simulink model "visualize_imu"  (Simulink 8.8)
settings: Solver=FixedStepDiscrete  StartTime=0.0  StopTime=inf  FixedStep=0.01  RelTol=1e-3  EnableMultiTasking=on
libraries: WBToolboxLibrary x2
settings Model: SuppressorTable=22 serialization::archive 11 0 3 0 0 0 11 0  Creator=The MathWorks, Inc.  LastModifiedBy=gnava
settings DataIOCC: SaveFormat=Dataset  SignalLoggingSaveFormat=Dataset
settings DebuggingCC: UnderspecifiedInitializationDetection=Simplified  MergeDetectMultiDrivingBlocksExec=error  FcnCallInpInsideContextMsg=error  AllowSymbolicDim=off  StateNameClashWarn=none
settings HardwareCC: ProdBitPerPointer=64  ProdBitPerSizeT=64  ProdBitPerPtrDiffT=64  ProdLargestAtomicFloat=Float  ProdIntDivRoundTo=Zero  ProdEndianess=LittleEndian  ProdWordSize=64  ProdHWDeviceType=Intel->x86-64 (Windows64)
settings GRTTargetCC: GeneratePreprocessorConditionals=Use local settings  CombineOutputUpdateFcns=on  GRTInterface=off

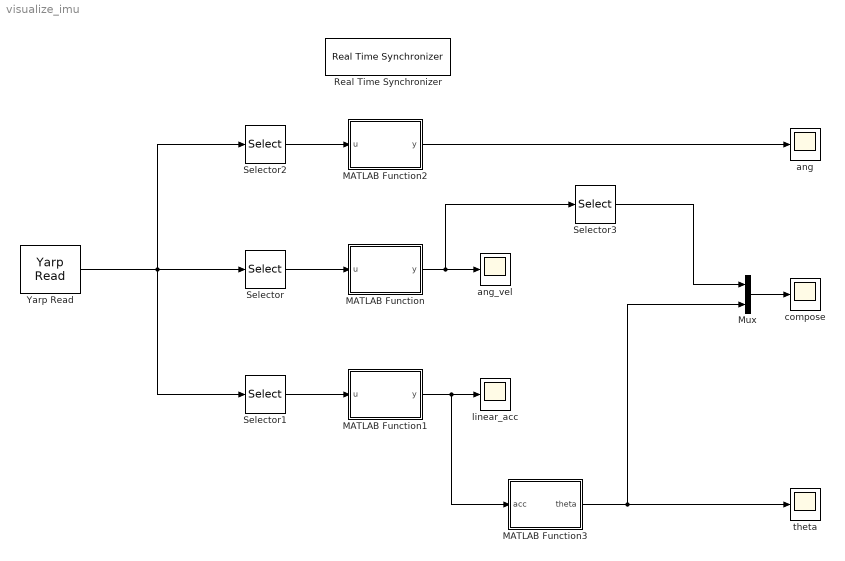
== system visualize_imu ==
  MATLAB Function : MATLAB Function  TreatAsAtomicUnit=on
  MATLAB Function1 : MATLAB Function  TreatAsAtomicUnit=on
  MATLAB Function2 : MATLAB Function  TreatAsAtomicUnit=on
  MATLAB Function3 : MATLAB Function  TreatAsAtomicUnit=on
  Mux : Mux  Inputs=2
  Real Time Synchronizer : WBToolboxLibrary/Utilities/Real Time Synchronizer  period=0.01
  Selector : Selector  InputPortWidth=9  IndexOptions=Index vector (dialog)  Indices=[7 8 9]  OutputSizes=1
  Selector1 : Selector  InputPortWidth=9  IndexOptions=Index vector (dialog)  Indices=[4 5 6]  OutputSizes=1
  Selector2 : Selector  InputPortWidth=9  IndexOptions=Index vector (dialog)  Indices=[1 2 3]  OutputSizes=1
  Selector3 : Selector  InputPortWidth=3  IndexOptions=Index vector (dialog)  Indices=[1]  OutputSizes=1
  Yarp Read : WBToolboxLibrary/Utilities/Yarp Read  portName='/seesaw'  signalSize=9  blocking=off  timestamp=off  autoconnect=on  errorOnConnection=on
  ang : Scope
  ang_vel : Scope
  compose : Scope
  linear_acc : Scope
  theta : Scope
  wires:
  Yarp Read/1 -> Selector1/1, Selector2/1, Selector/1
  Selector/1 -> MATLAB Function/1(u)
  MATLAB Function/1(y) -> Selector3/1, ang_vel/1
  Selector1/1 -> MATLAB Function1/1(u)
  MATLAB Function1/1(y) -> MATLAB Function3/1(acc), linear_acc/1
  Selector2/1 -> MATLAB Function2/1(u)
  MATLAB Function2/1(y) -> ang/1
  MATLAB Function3/1(theta) -> Mux/2, theta/1
  Selector3/1 -> Mux/1
  Mux/1 -> compose/1

== matlab function MATLAB Function1 ==
  data: u input double; y output double
function y = rotate(u)

y = rotx(pi)*rotz(-44/180*pi)*u;

== matlab function MATLAB Function ==
  data: u input double; y output double
function y = rotate(u)

y = rotx(pi)*rotz(-44/180*pi)*u;

== matlab function MATLAB Function2 ==
  data: u input double; y output double
function y = rotate(u)

y = rotx(pi)*rotz(-44/180*pi)*u;

== matlab function MATLAB Function3 ==
  data: acc input double; theta output double
function theta = arctangent(acc)

theta = atan2(acc(2),acc(3))*180/pi;

end
